simulink model "simulation_with_sensors"  (R2023b)
settings: Solver=VariableStepAuto  StartTime=0.0  StopTime=1000  RelTol=1e-3
values from neighbouring files (symbols this model uses):
  a = R_E+500*1e3    (= 6871000)    [Sensors.m]    (also in sim_with_sensors.m = 6851.22197053; simulation_with_sensors.m = 26584)
  A_313 = ( R_om * R_i * R_OM )'    [simulation_with_sensors.m]
  e = 0    [Sensors.m]    (also in sim_with_sensors.m = 0.00183012221618; simulation_with_sensors.m = 0.00023103)
  H0 = sqrt(g01^2+g11^2+h11^2)*1e-9    [sim_with_sensors.m]    (also in simulation_with_sensors.m)
  I = diag([I1 I2 I3])*1e-9    [sim_with_sensors.m]    (also in simulation_with_sensors.m = diag([100.09 25.1 91.6]))
  i = 1.699980862034725    (= 1.69998086203)    [sim_with_sensors.m]    (also in simulation_with_sensors.m = 0.9601)
  I_inv = inv(I)    [simulation_with_sensors.m]
  incl = deg2rad(11.5)    [sim_with_sensors.m]    (also in simulation_with_sensors.m)
  n = n+1    (= 1)    [Sensors.m]    (also in sim_with_sensors.m = sqrt(mu/a^3); simulation_with_sensors.m = sqrt(astroConstants(13) / a^3))
  omegaE = deg2rad(15)/3600    [sim_with_sensors.m]    (also in simulation_with_sensors.m)
  P = zeros(lenn,lenm)    [Sensors.m]
  s0 = zeros(3,1)    [sim_with_sensors.m]    (also in simulation_with_sensors.m = [0; 0; 0])
  tol = 1e-2    (= 0.01)    [simulation_with_sensors.m]
  w0 = [0.2; 0; 0.2]    [simulation_with_sensors.m]
undefined symbols (not defined in the file or in its folder): A, c1, magnitude, N, n_sun, onesM, onesV, r_Fskew, rho_d, rho_s
libraries: matrix_library x11, dspmathops x10, simulink x3
(part 1 of 2)
settings Model: Creator=danie  LastModifiedBy=danie

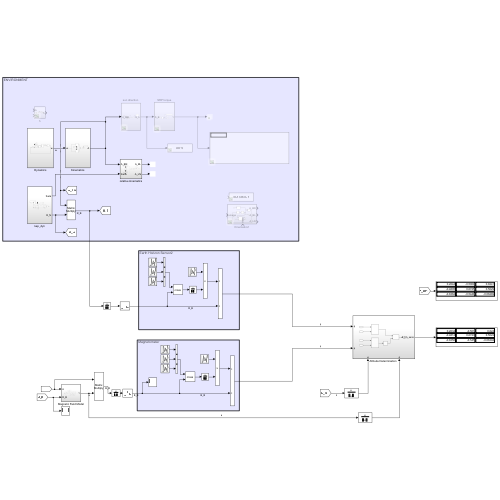
[thumbnail: Simulink's stored preview of the top-level diagram]
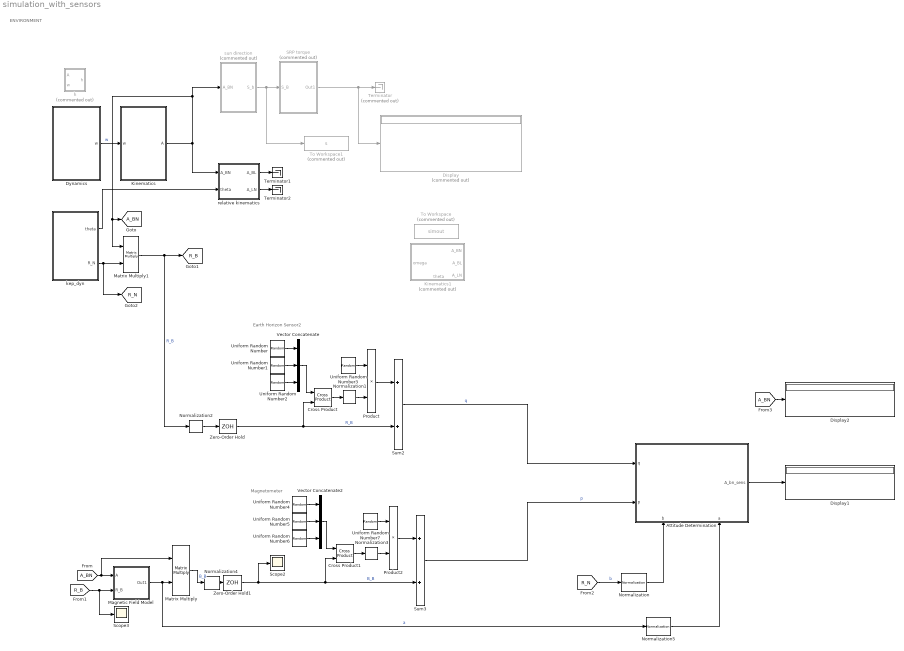
== system simulation_with_sensors ==
  note: ENVIRONMENT
  note: Earth Horizon Sensor2
  note: Magnetometer
  "Attitude Determination  " : Subsystem
      settings: PortSchema="{\"entries\":[{\"content\":{\"sides\":[{\"content\":{\"connectorIds\":[\"In1\",\"In2\"]},\"type\":\"ConnectorPlacement.EquallySpacedRectSide\",\"uuid\":\"730966cf-d0d7-44a0-92f0-b5324480e7cc\"},{\"content\":{\"connectorIds\":[\"Out1\"],\"side\":\"RIGHT\"},\"type\":\"ConnectorPlacement.EquallySpacedRectSide\",\"uuid\":\"c83e6b57-46fe-4a45-9824-d3495e15bf6a\"},{\"content\":{\"side\":\"TOP\"},\"type\":\"ConnectorPlacement.EquallySpacedRectSide\",\"uuid\":\"4938c298-c2b3-45b7-bcb0-70b8132dabc6\"},{\"content\":{\"connectorIds\":[\"In3\",\"In4\"],\"side\":\"BOTTOM\"},\"type\":\"ConnectorPlacement.EquallySpacedRectSide\",\"uuid\":\"6d6a244e-80db-423b-a0a5-9a5face48fcb\"}]},\"type\":\"ConnectorPlacement.EquallySpacedConnector\",\"uuid\":\"7eb6767d-3ff0-4577-86c9-ebc5e763f220\"}],\"packageUris\":[\"http://schema.mathworks.com/mf0/Connector/R2020b\"],\"version\":\"1.0\"}"
  Cross Product : matrix_library/Cross Product
  Cross Product1 : matrix_library/Cross Product
  Display : Display  Commented=on
  Display1 : Display
  Display2 : Display
  Dynamics : Subsystem
  Kinematics : Subsystem
  Kinematics1 : Subsystem  Commented=on
      settings: PortSchema="{\"entries\":[{\"content\":{\"sides\":[{\"content\":{\"connectorIds\":[\"In1\"]},\"type\":\"ConnectorPlacement.EquallySpacedRectSide\",\"uuid\":\"c78567b3-0f16-47a3-80bd-0d4e0067a31f\"},{\"content\":{\"connectorIds\":[\"Out1\",\"Out2\",\"Out3\"],\"side\":\"RIGHT\"},\"type\":\"ConnectorPlacement.EquallySpacedRectSide\",\"uuid\":\"73465dec-5215-44e7-a1cc-75f9f3cf9a64\"},{\"content\":{\"side\":\"TOP\"},\"type\":\"ConnectorPlacement.EquallySpacedRectSide\",\"uuid\":\"3a97d62b-3b72-49ee-88a3-b4c3b7bde741\"},{\"content\":{\"connectorIds\":[\"In2\"],\"side\":\"BOTTOM\"},\"type\":\"ConnectorPlacement.EquallySpacedRectSide\",\"uuid\":\"877f870a-38cc-42df-9514-c8e95f578485\"}]},\"type\":\"ConnectorPlacement.EquallySpacedConnector\",\"uuid\":\"7c502635-8079-4510-841d-e1e17271f078\"}],\"packageUris\":[\"http://schema.mathworks.com/mf0/Connector/R2020b\"],\"version\":\"1.0\"}"
  Magnetic Field Model : Subsystem
  Matrix Multiply : Product  Multiplication=Matrix(*)
  Matrix Multiply1 : Product  Multiplication=Matrix(*)
  Normalization{,1..5} (6 alike) : dspmathops/Normalization  NormType=2-norm  Bias=1e-10  NormOver=Each column  Dimension=1  roundingMode=Floor  overflowMode=off  accumDataTypeStr=Inherit: Same as product output  accumLastDataTypeStr=Inherit: Same as product output  outputDataTypeStr=Inherit: Same as product output  outputMin=[]  outputMax=[]  outputLastDataTypeStr=Inherit: Same as product output
  Product : Product
  Product2 : Product
  SRP torque : Subsystem  Commented=on
  Scope2 : Scope
  Scope3 : Scope
  Sum2 : Sum
  Sum3 : Sum
  Terminator : Terminator  Commented=on
  Terminator1 : Terminator
  Terminator2 : Terminator
  To Workspace : ToWorkspace  Commented=on  VariableName=simout  SaveFormat=Timeseries  SampleTime=-1
  To Workspace1 : ToWorkspace  Commented=on  VariableName=s  SaveFormat=Timeseries  SampleTime=-1
  Uniform Random Number{,1..2,4..6} (6 alike) : UniformRandomNumber
  Uniform Random Number3 : UniformRandomNumber  Minimum=0  Maximum=tan(deg2rad(0.1))
  Uniform Random Number7 : UniformRandomNumber  Minimum=0  Maximum=tan(deg2rad(0.5))
  Vector Concatenate : Concatenate  NumInputs=3
  Vector Concatenate2 : Concatenate  NumInputs=3
  Zero-Order Hold : ZeroOrderHold  SampleTime=1/30
  Zero-Order Hold1 : ZeroOrderHold  SampleTime=1/30
  h : Subsystem  Commented=on
  kep_dyn : Subsystem
  relative kinematics : Subsystem
  "sun direction " : Subsystem  Commented=on
  tag scope: A_BN=global, R_B=global, R_N=global
  wires:
  kep_dyn/2(R_N) -> [R_N], Matrix Multiply1/2
  SRP torque/1(Out1) -> Display/1, Terminator/1
  Dynamics/1(w) -> Kinematics/1(w)  "w"
  "sun direction "/1(S_b) -> SRP torque/1(S_B), To Workspace1/1
  Kinematics/1(A) -> [A_BN], Matrix Multiply1/1, "sun direction "/1(A_BN), relative kinematics/1(A_BN)
  kep_dyn/1(theta) -> relative kinematics/2(theta)
  Sum2/1 -> "Attitude Determination  "/1(q)  "q"
  Normalization1/1 -> Product/2
  Magnetic Field Model/1(Out1) -> Normalization5/1, Matrix Multiply/2  "a"
  Uniform Random Number3/1 -> Product/1
  Uniform Random Number7/1 -> Product2/1
  Uniform Random Number1/1 -> Vector Concatenate/2
  Uniform Random Number5/1 -> Vector Concatenate2/2
  Uniform Random Number4/1 -> Vector Concatenate2/1
  Product/1 -> Sum2/1
  Product2/1 -> Sum3/1
  Zero-Order Hold1/1 -> Cross Product1/2, Sum3/2, Scope2/1  "B_B"
  Vector Concatenate2/1 -> Cross Product1/1
  Normalization3/1 -> Product2/2
  Sum3/1 -> "Attitude Determination  "/2(p)  "p"
  Cross Product1/1 -> Normalization3/1
  Normalization2/1 -> Zero-Order Hold/1
  Zero-Order Hold/1 -> Cross Product/2, Sum2/2  "R_B"
  Uniform Random Number/1 -> Vector Concatenate/1
  Vector Concatenate/1 -> Cross Product/1
  Uniform Random Number2/1 -> Vector Concatenate/3
  Uniform Random Number6/1 -> Vector Concatenate2/3
  Cross Product/1 -> Normalization1/1
  Matrix Multiply1/1 -> [R_B], Normalization2/1  "R_B"
  [A_BN] -> Matrix Multiply/1, Magnetic Field Model/1(A)
  [R_B] -> Scope3/1, Magnetic Field Model/2(R_B)
  relative kinematics/1(A_BL) -> Terminator1/1
  relative kinematics/2(A_LN) -> Terminator2/1
  Normalization4/1 -> Zero-Order Hold1/1
  Matrix Multiply/1 -> Normalization4/1  "B_B"
  [R_N] -> Normalization/1  "b"
  "Attitude Determination  "/1(A_bn_sens) -> Display1/1
  [A_BN] -> Display2/1
  Normalization/1 -> "Attitude Determination  "/3(b)
  Normalization5/1 -> "Attitude Determination  "/4(a)

== system simulation_with_sensors/Attitude Determination   ==
  q : Inport
  p : Inport  Port=2
  b : Inport  Port=3
  a : Inport  Port=4
  Matrix Multiply : Product  Multiplication=Matrix(*)
  S : Subsystem
  Transpose : Math  Operator=transpose
  V : Subsystem
  A_bn_sens : Outport
  wires:
  q/1 -> S/1(q)
  p/1 -> S/2(p)
  a/1 -> V/2(a)
  b/1 -> V/1(b)
  V/1(V) -> Transpose/1
  S/1(S) -> Matrix Multiply/1
  Transpose/1 -> Matrix Multiply/2
  Matrix Multiply/1 -> A_bn_sens/1

== system simulation_with_sensors/Dynamics ==
  Constant : Constant  Value=I
  Constant1 : Constant  Value=-I_inv
  Cross Product : matrix_library/Cross Product
  Integrator : Integrator  InitialCondition=w0
  Product : Product  Multiplication=Matrix(*)
  Product1 : Product  Multiplication=Matrix(*)
  To Workspace : ToWorkspace  VariableName=w  SaveFormat=Timeseries  SampleTime=-1
  w : Outport
  wires:
  Cross Product/1 -> Product1/2
  Constant/1 -> Product/1
  Integrator/1 -> Product/2, w/1, To Workspace/1, Cross Product/1  "w"
  Constant1/1 -> Product1/1
  Product/1 -> Cross Product/2
  Product1/1 -> Integrator/1  "wdot"

== system simulation_with_sensors/Kinematics ==
  w : Inport
  Kinematics 312 : Subsystem
  Kinematics 313 : Subsystem
  Merge : Merge
  NOT : Logic  Operator=NOT  IconShape=distinctive  AllPortsSameDT=off  OutDataTypeStr=boolean
  System switcher : Subsystem
  To Workspace : ToWorkspace  VariableName=A  SaveFormat=Timeseries  SampleTime=-1
  A : Outport
  wires:
  NOT/1 -> Kinematics 313/Enable
  w/1 -> Kinematics 312/1(w), Kinematics 313/1(w)
  System switcher/1(flag) -> Kinematics 312/Enable, NOT/1
  Kinematics 313/1(A) -> Merge/2
  Merge/1 -> A/1, To Workspace/1  "A"
  Kinematics 312/1(A) -> Merge/1

== system simulation_with_sensors/Kinematics1 ==
  omega : Inport
  theta : Inport  Port=2
  Integrator : Integrator  InitialCondition=eye(3)
  Matrix Multiply : Product  Multiplication=Matrix(*)
  om^ : Subsystem
  orthonormalization1 : Subsystem
  relative kinematics : Subsystem
  A_BN : Outport
  A_BL : Outport  Port=2
  A_LN : Outport  Port=3
  wires:
  Integrator/1 -> orthonormalization1/1(A0)
  omega/1 -> om^/1(omega)
  om^/1(" om ^") -> Matrix Multiply/1
  Matrix Multiply/1 -> Integrator/1
  orthonormalization1/1(A) -> relative kinematics/1(A_BN), A_BN/1, Matrix Multiply/2
  relative kinematics/1(A_BL) -> A_BL/1
  theta/1 -> relative kinematics/2(theta)
  relative kinematics/2(A_LN) -> A_LN/1

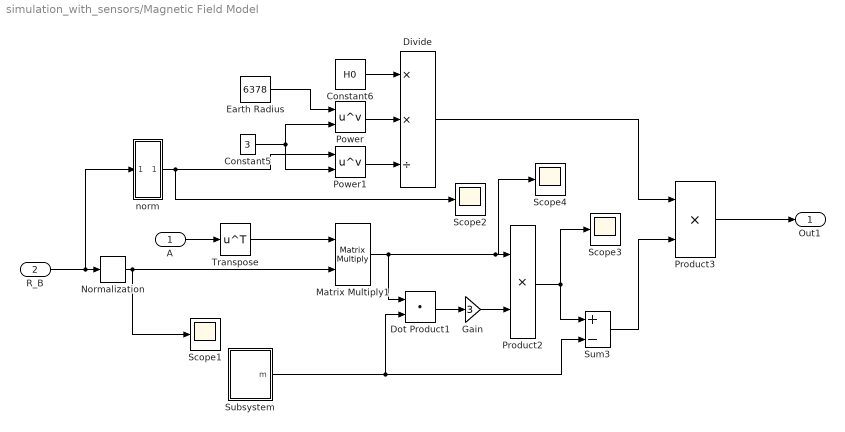
== system simulation_with_sensors/Magnetic Field Model ==
  A : Inport
  R_B : Inport  Port=2
  Constant5 : Constant  Value=3
  Constant6 : Constant  Value=H0
  Divide : Product  Inputs=**/
  Dot Product1 : DotProduct  OutDataTypeStr=Inherit: Inherit via internal rule
  Earth Radius : Constant  Value=6378
  Gain : Gain  Gain=3
  Matrix Multiply1 : Product  Multiplication=Matrix(*)
  Normalization : dspmathops/Normalization  NormType=2-norm  Bias=1e-10  NormOver=Each column  Dimension=1  roundingMode=Floor  overflowMode=off  accumDataTypeStr=Inherit: Same as product output  accumLastDataTypeStr=Inherit: Same as product output  outputDataTypeStr=Inherit: Same as product output  outputMin=[]  outputMax=[]  outputLastDataTypeStr=Inherit: Same as product output
  Power : Math  Operator=pow
  Power1 : Math  Operator=pow
  Product2 : Product
  Product3 : Product
  Scope{1..4} (4 alike) : Scope
  Subsystem : Subsystem
  Sum3 : Sum  Inputs=+-
  Transpose : Math  Operator=transpose
  norm : Subsystem
  Out1 : Outport
  wires:
  Matrix Multiply1/1 -> Scope4/1, Product2/1, Dot Product1/1
  Subsystem/1(m) -> Sum3/2, Dot Product1/2
  R_B/1 -> norm/1(In1), Normalization/1
  Divide/1 -> Product3/1
  Constant5/1 -> Power/2, Power1/2
  Sum3/1 -> Product3/2
  norm/1(Out1) -> Scope2/1, Power1/1
  Dot Product1/1 -> Gain/1
  Gain/1 -> Product2/2
  Product2/1 -> Sum3/1, Scope3/1
  Earth Radius/1 -> Power/1
  Constant6/1 -> Divide/1
  Transpose/1 -> Matrix Multiply1/1
  Power/1 -> Divide/2
  A/1 -> Transpose/1
  Product3/1 -> Out1/1
  Power1/1 -> Divide/3
  Normalization/1 -> Scope1/1, Matrix Multiply1/2

== system simulation_with_sensors/SRP torque ==
  S_B : Inport
  Display : Display
  SRP forces calc : Subsystem
  To Workspace : ToWorkspace  VariableName=SRP_F  SaveFormat=Timeseries  SampleTime=-1
  To Workspace1 : ToWorkspace  VariableName=SRP_T  SaveFormat=Timeseries  SampleTime=-1
  equivalent force system : Subsystem
  Out1 : Outport
  wires:
  equivalent force system/1(Torque) -> Display/1, To Workspace1/1, Out1/1
  equivalent force system/2(Resultant) -> To Workspace/1
  S_B/1 -> SRP forces calc/1(In1)  "SUN DIR."
  SRP forces calc/1(forces) -> equivalent force system/1(Forces)

== system simulation_with_sensors/h ==
  A : Inport
  w : Inport  Port=2
  Constant : Constant  Value=I
  Product1 : Product  Multiplication=Matrix(*)
  Product2 : Product  Multiplication=Matrix(*)
  Transpose : Math  Operator=transpose
  h : Outport
  wires:
  Constant/1 -> Product1/1
  Product2/1 -> h/1  "h"
  Product1/1 -> Product2/2  "h_body"
  A/1 -> Transpose/1
  w/1 -> Product1/2
  Transpose/1 -> Product2/1

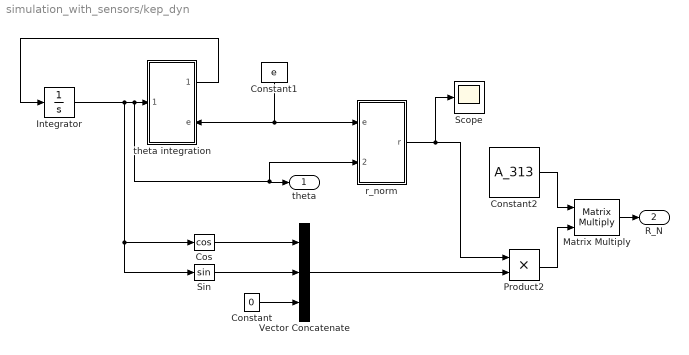
== system simulation_with_sensors/kep_dyn ==
  Constant : Constant  Value=0
  Constant1 : Constant  Value=e
  Constant2 : Constant  Value=A_313
  Cos : Trigonometry  Operator=cos
  Integrator : Integrator
  Matrix Multiply : Product  Multiplication=Matrix(*)
  Product2 : Product
  Scope : Scope
  Sin : Trigonometry
  Vector Concatenate : Concatenate  NumInputs=3
  r_norm : Subsystem
  theta integration : Subsystem
      settings: PortSchema="{\"entries\":[{\"content\":{\"sides\":[{\"content\":{\"connectorIds\":[\"In1\"]},\"type\":\"ConnectorPlacement.EquallySpacedRectSide\",\"uuid\":\"3f1b1ec9-07ed-4eb1-9e41-630dc5613e97\"},{\"content\":{\"connectorIds\":[\"Out1\",\"In2\"],\"side\":\"RIGHT\"},\"type\":\"ConnectorPlacement.EquallySpacedRectSide\",\"uuid\":\"22d0f7bc-714c-4365-a26c-07047ff4be14\"},{\"content\":{\"side\":\"TOP\"},\"type\":\"ConnectorPlacement.EquallySpacedRectSide\",\"uuid\":\"875f7006-d698-4730-93ae-1a7d05f24054\"}]},\"type\":\"ConnectorPlacement.EquallySpacedConnector\",\"uuid\":\"799b65b1-faea-432b-9f3f-2d21984184cd\"}],\"packageUris\":[\"http://schema.mathworks.com/mf0/Connector/R2020b\"],\"version\":\"1.0\"}"
  theta : Outport
  R_N : Outport  Port=2
  wires:
  Integrator/1 -> Sin/1, Cos/1, r_norm/2(theta), theta/1, theta integration/1(theta)
  theta integration/1(theta_dot) -> Integrator/1
  Constant/1 -> Vector Concatenate/3
  Cos/1 -> Vector Concatenate/1
  Constant1/1 -> theta integration/2(e), r_norm/1(e)
  r_norm/1(r) -> Scope/1, Product2/1
  Vector Concatenate/1 -> Product2/2
  Sin/1 -> Vector Concatenate/2
  Constant2/1 -> Matrix Multiply/1
  Product2/1 -> Matrix Multiply/2
  Matrix Multiply/1 -> R_N/1

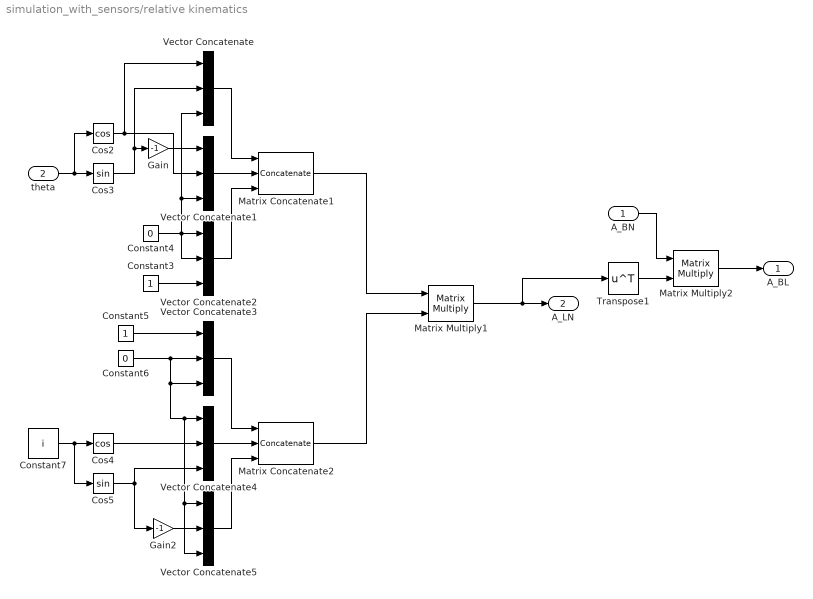
== system simulation_with_sensors/relative kinematics ==
  A_BN : Inport
  theta : Inport  Port=2
  Constant3 : Constant
  Constant4 : Constant  Value=0
  Constant5 : Constant
  Constant6 : Constant  Value=0
  Constant7 : Constant  Value=i
  Cos2 : Trigonometry  Operator=cos
  Cos3 : Trigonometry
  Cos4 : Trigonometry  Operator=cos
  Cos5 : Trigonometry
  Gain : Gain  Gain=-1
  Gain2 : Gain  Gain=-1
  Matrix Concatenate1 : Concatenate  NumInputs=3  Mode=Multidimensional array  ConcatenateDimension=2
  Matrix Concatenate2 : Concatenate  NumInputs=3  Mode=Multidimensional array  ConcatenateDimension=2
  Matrix Multiply1 : Product  Multiplication=Matrix(*)
  Matrix Multiply2 : Product  Multiplication=Matrix(*)
  Transpose1 : Math  Operator=transpose
  Vector Concatenate{,1..5} (6 alike) : Concatenate  NumInputs=3
  A_BL : Outport
  A_LN : Outport  Port=2
  wires:
  Cos2/1 -> Vector Concatenate1/2, Vector Concatenate/1
  Cos3/1 -> Gain/1, Vector Concatenate/2
  Constant4/1 -> Vector Concatenate2/2, Vector Concatenate/3, Vector Concatenate1/3, Vector Concatenate2/1
  Constant3/1 -> Vector Concatenate2/3
  Gain/1 -> Vector Concatenate1/1
  theta/1 -> Cos2/1, Cos3/1
  Vector Concatenate/1 -> Matrix Concatenate1/1
  Vector Concatenate1/1 -> Matrix Concatenate1/2
  Vector Concatenate2/1 -> Matrix Concatenate1/3
  Vector Concatenate5/1 -> Matrix Concatenate2/3
  Constant7/1 -> Cos4/1, Cos5/1
  Vector Concatenate3/1 -> Matrix Concatenate2/1
  Cos5/1 -> Vector Concatenate4/3, Gain2/1
  Vector Concatenate4/1 -> Matrix Concatenate2/2
  Constant5/1 -> Vector Concatenate3/1
  Constant6/1 -> Vector Concatenate5/3, Vector Concatenate5/1, Vector Concatenate4/1, Vector Concatenate3/3, Vector Concatenate3/2
  Cos4/1 -> Vector Concatenate4/2
  Gain2/1 -> Vector Concatenate5/2
  Matrix Concatenate1/1 -> Matrix Multiply1/1
  Matrix Concatenate2/1 -> Matrix Multiply1/2
  Matrix Multiply1/1 -> Transpose1/1, A_LN/1
  A_BN/1 -> Matrix Multiply2/1
  Transpose1/1 -> Matrix Multiply2/2
  Matrix Multiply2/1 -> A_BL/1

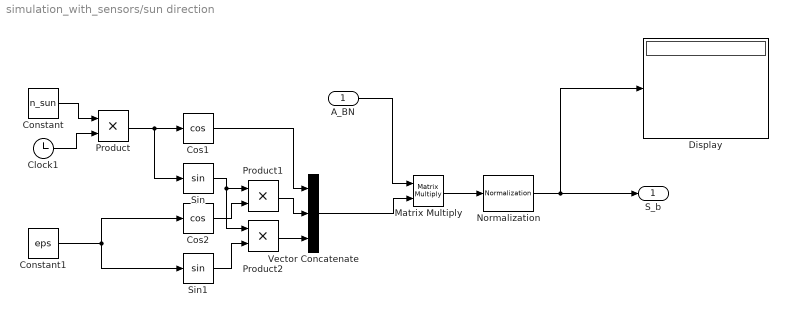
== system simulation_with_sensors/sun direction  ==
  A_BN : Inport
  Clock1 : Clock
  Constant : Constant  Value=n_sun
  Constant1 : Constant  Value=eps
  Cos1 : Trigonometry  Operator=cos
  Cos2 : Trigonometry  Operator=cos
  Display : Display
  Matrix Multiply : Product  Multiplication=Matrix(*)
  Normalization : dspmathops/Normalization  NormType=Squared 2-norm  Bias=1e-10  NormOver=Each column  Dimension=1  roundingMode=Floor  overflowMode=off  accumDataTypeStr=Inherit: Same as product output  accumLastDataTypeStr=Inherit: Same as product output  outputDataTypeStr=Inherit: Same as product output  outputMin=[]  outputMax=[]  outputLastDataTypeStr=Inherit: Same as product output
  Product : Product
  Product1 : Product
  Product2 : Product
  Sin : Trigonometry
  Sin1 : Trigonometry
  Vector Concatenate : Concatenate  NumInputs=3
  S_b : Outport
  wires:
  Constant/1 -> Product/1
  Clock1/1 -> Product/2
  Product/1 -> Sin/1, Cos1/1
  Constant1/1 -> Sin1/1, Cos2/1
  Sin/1 -> Product2/1, Product1/1
  Cos2/1 -> Product1/2
  Sin1/1 -> Product2/2
  Cos1/1 -> Vector Concatenate/1
  Product1/1 -> Vector Concatenate/2
  Product2/1 -> Vector Concatenate/3
  Matrix Multiply/1 -> Normalization/1
  A_BN/1 -> Matrix Multiply/1
  Normalization/1 -> Display/1, S_b/1
  Vector Concatenate/1 -> Matrix Multiply/2

== system simulation_with_sensors/Attitude Determination  /S ==
  q : Inport
  p : Inport  Port=2
  Cross Product : matrix_library/Cross Product
  Cross Product1 : matrix_library/Cross Product
  Matrix Concatenate : Concatenate  NumInputs=3  Mode=Multidimensional array  ConcatenateDimension=2
  Normalization : dspmathops/Normalization  NormType=2-norm  Bias=1e-10  NormOver=Each column  Dimension=1  roundingMode=Floor  overflowMode=off  accumDataTypeStr=Inherit: Same as product output  accumLastDataTypeStr=Inherit: Same as product output  outputDataTypeStr=Inherit: Same as product output  outputMin=[]  outputMax=[]  outputLastDataTypeStr=Inherit: Same as product output
  S : Outport
  wires:
  p/1 -> Matrix Concatenate/1, Cross Product/1, Cross Product1/1
  q/1 -> Cross Product/2
  Cross Product/1 -> Normalization/1
  Normalization/1 -> Matrix Concatenate/2, Cross Product1/2
  Matrix Concatenate/1 -> S/1
  Cross Product1/1 -> Matrix Concatenate/3

== system simulation_with_sensors/Attitude Determination  /V ==
  b : Inport
  a : Inport  Port=2
  Cross Product : matrix_library/Cross Product
  Cross Product1 : matrix_library/Cross Product
  Matrix Concatenate : Concatenate  NumInputs=3  Mode=Multidimensional array  ConcatenateDimension=2
  Normalization : dspmathops/Normalization  NormType=2-norm  Bias=1e-10  NormOver=Each column  Dimension=1  roundingMode=Floor  overflowMode=off  accumDataTypeStr=Inherit: Same as product output  accumLastDataTypeStr=Inherit: Same as product output  outputDataTypeStr=Inherit: Same as product output  outputMin=[]  outputMax=[]  outputLastDataTypeStr=Inherit: Same as product output
  V : Outport
  wires:
  Cross Product1/1 -> Matrix Concatenate/3
  Matrix Concatenate/1 -> V/1
  Normalization/1 -> Cross Product1/2, Matrix Concatenate/2
  Cross Product/1 -> Normalization/1
  b/1 -> Cross Product/2
  a/1 -> Cross Product1/1, Cross Product/1, Matrix Concatenate/1

== system simulation_with_sensors/Kinematics/Kinematics 312 ==
  w : Inport
  Enable : EnablePort  StatesWhenEnabling=reset
  A - s_312 : Subsystem
  Euler angles : Subsystem
  IC : InitialCondition  Value=s0
  s_312 - A : Subsystem
  s_313 - A : Subsystem
  A : Outport
  wires:
  s_312 - A/1(A) -> A/1  "A"
  Euler angles/1(s) -> s_312 - A/1(s)  "s"
  w/1 -> Euler angles/1(w)
  IC/1 -> Euler angles/2(s0)
  A - s_312/1(s) -> IC/1
  s_313 - A/1(A) -> A - s_312/1(A)
  [s_313] -> s_313 - A/1(s)

== system simulation_with_sensors/Kinematics/Kinematics 313 ==
  w : Inport
  Enable : EnablePort  StatesWhenEnabling=reset
  A - s_313 : Subsystem
  Euler angles : Subsystem
  s_312 - A : Subsystem
  s_313 - A : Subsystem
  A : Outport
  wires:
  w/1 -> Euler angles/1(w)
  Euler angles/1(s) -> s_313 - A/1(s)
  s_313 - A/1(A) -> A/1
  A - s_313/1(s) -> Euler angles/2(s0)
  s_312 - A/1(A) -> A - s_313/1(A)
  [s_312] -> s_312 - A/1(s)

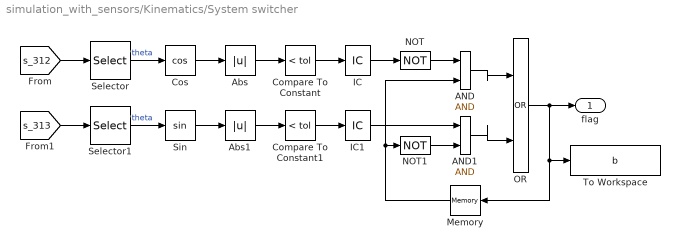
== system simulation_with_sensors/Kinematics/System switcher ==
  AND : Logic  IconShape=distinctive  AllPortsSameDT=off  OutDataTypeStr=boolean
  AND1 : Logic  IconShape=distinctive  AllPortsSameDT=off  OutDataTypeStr=boolean
  Abs : Abs  SaturateOnIntegerOverflow=off
  Abs1 : Abs  SaturateOnIntegerOverflow=off
  Compare To Constant : simulink/Logic and Bit Operations/Compare To Constant  relop=<  const=tol  OutDataTypeStr=boolean
  Compare To Constant1 : simulink/Logic and Bit Operations/Compare To Constant  relop=<  const=tol  OutDataTypeStr=boolean
  Cos : Trigonometry  Operator=cos
  IC : InitialCondition  Value=0
  IC1 : InitialCondition  Value=0
  Memory : Memory  InitialCondition=1
  NOT : Logic  Operator=NOT  IconShape=distinctive  AllPortsSameDT=off  OutDataTypeStr=boolean
  NOT1 : Logic  Operator=NOT  IconShape=distinctive  AllPortsSameDT=off  OutDataTypeStr=boolean
  OR : Logic  Operator=OR  IconShape=distinctive  AllPortsSameDT=off  OutDataTypeStr=boolean
  Selector : Selector  InputPortWidth=3  IndexOptions=Index vector (dialog)  Indices=2  OutputSizes=1
  Selector1 : Selector  InputPortWidth=3  IndexOptions=Index vector (dialog)  Indices=2  OutputSizes=1
  Sin : Trigonometry
  To Workspace : ToWorkspace  VariableName=b  SaveFormat=Timeseries  SampleTime=-1
  flag : Outport
  wires:
  Cos/1 -> Abs/1
  [s_312] -> Selector/1
  Compare To Constant/1 -> IC/1
  Selector1/1 -> Sin/1  "theta"
  Abs/1 -> Compare To Constant/1
  Compare To Constant1/1 -> IC1/1
  Selector/1 -> Cos/1  "theta"
  Abs1/1 -> Compare To Constant1/1
  Sin/1 -> Abs1/1
  [s_313] -> Selector1/1
  IC/1 -> NOT/1
  NOT/1 -> AND/1
  AND/1 -> OR/1
  NOT1/1 -> AND1/2
  IC1/1 -> AND1/1
  AND1/1 -> OR/2
  OR/1 -> To Workspace/1, Memory/1, flag/1
  Memory/1 -> AND/2, NOT1/1

== system simulation_with_sensors/Kinematics1/om^ ==
  omega : Inport
  Constant : Constant  Value=[1; 0; 0]
  Constant1 : Constant  Value=[0; 1; 0]
  Constant2 : Constant  Value=[0; 0; 1]
  Cross Product : matrix_library/Cross Product
  Cross Product1 : matrix_library/Cross Product
  Cross Product2 : matrix_library/Cross Product
  Matrix Concatenate : Concatenate  NumInputs=3  Mode=Multidimensional array  ConcatenateDimension=2
  " om ^" : Outport
  wires:
  Matrix Concatenate/1 -> " om ^"/1
  Cross Product2/1 -> Matrix Concatenate/3
  Cross Product1/1 -> Matrix Concatenate/2
  Cross Product/1 -> Matrix Concatenate/1
  Constant/1 -> Cross Product/1
  Constant1/1 -> Cross Product1/1
  Constant2/1 -> Cross Product2/1
  omega/1 -> Cross Product/2, Cross Product1/2, Cross Product2/2

== system simulation_with_sensors/Kinematics1/orthonormalization1 ==
  A0 : Inport
  Gain : Gain  Gain=3/2
  Gain1 : Gain  Gain=1/2
  Matrix Multiply : Product  Inputs=3  Multiplication=Matrix(*)
  Sum : Sum  Inputs=-|+
  Transpose : matrix_library/Transpose
  A : Outport
  wires:
  Sum/1 -> A/1
  Gain1/1 -> Sum/1
  Matrix Multiply/1 -> Gain1/1
  Transpose/1 -> Matrix Multiply/2
  Gain/1 -> Sum/2
  A0/1 -> Gain/1, Matrix Multiply/3, Transpose/1, Matrix Multiply/1

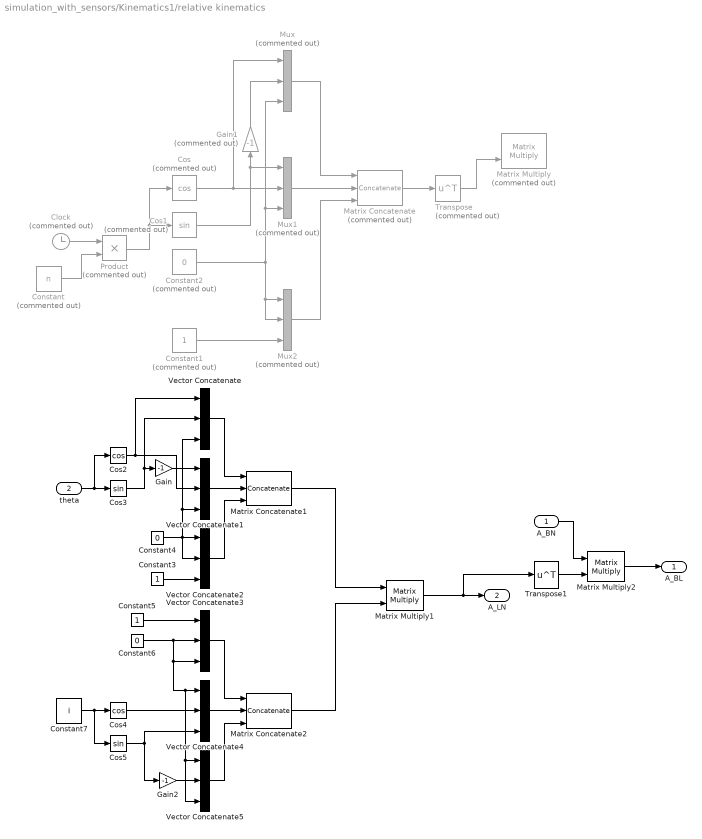
== system simulation_with_sensors/Kinematics1/relative kinematics ==
  A_BN : Inport
  theta : Inport  Port=2
  Clock : Clock  Commented=on
  Constant : Constant  Commented=on  Value=n
  Constant1 : Constant  Commented=on
  Constant2 : Constant  Commented=on  Value=0
  Constant3 : Constant
  Constant4 : Constant  Value=0
  Constant5 : Constant
  Constant6 : Constant  Value=0
  Constant7 : Constant  Value=i
  Cos : Trigonometry  Commented=on  Operator=cos
  Cos1 : Trigonometry  Commented=on
  Cos2 : Trigonometry  Operator=cos
  Cos3 : Trigonometry
  Cos4 : Trigonometry  Operator=cos
  Cos5 : Trigonometry
  Gain : Gain  Gain=-1
  Gain1 : Gain  Commented=on  Gain=-1
  Gain2 : Gain  Gain=-1
  Matrix Concatenate : Concatenate  Commented=on  NumInputs=3  Mode=Multidimensional array  ConcatenateDimension=2
  Matrix Concatenate1 : Concatenate  NumInputs=3  Mode=Multidimensional array  ConcatenateDimension=2
  Matrix Concatenate2 : Concatenate  NumInputs=3  Mode=Multidimensional array  ConcatenateDimension=2
  Matrix Multiply : Product  Commented=on  Multiplication=Matrix(*)
  Matrix Multiply1 : Product  Multiplication=Matrix(*)
  Matrix Multiply2 : Product  Multiplication=Matrix(*)
  Mux : Mux  Commented=on  Inputs=3
  Mux1 : Mux  Commented=on  Inputs=3
  Mux2 : Mux  Commented=on  Inputs=3
  Product : Product  Commented=on
  Transpose : Math  Commented=on  Operator=transpose
  Transpose1 : Math  Operator=transpose
  Vector Concatenate{,1..5} (6 alike) : Concatenate  NumInputs=3
  A_BL : Outport
  A_LN : Outport  Port=2
  wires:
  Product/1 -> Cos1/1, Cos/1
  Cos/1 -> Mux1/2, Mux/1
  Cos1/1 -> Gain1/1, Mux1/1
  Constant2/1 -> Mux1/3, Mux/3, Mux2/2, Mux2/1
  Gain1/1 -> Mux/2
  Constant1/1 -> Mux2/3
  Mux/1 -> Matrix Concatenate/1
  Mux1/1 -> Matrix Concatenate/2
  Mux2/1 -> Matrix Concatenate/3
  Matrix Concatenate/1 -> Transpose/1
  Transpose/1 -> Matrix Multiply/2
  Clock/1 -> Product/1
  Constant/1 -> Product/2
  Cos2/1 -> Vector Concatenate1/2, Vector Concatenate/1
  Cos3/1 -> Gain/1, Vector Concatenate/2
  Constant4/1 -> Vector Concatenate2/2, Vector Concatenate/3, Vector Concatenate1/3, Vector Concatenate2/1
  Constant3/1 -> Vector Concatenate2/3
  Gain/1 -> Vector Concatenate1/1
  theta/1 -> Cos2/1, Cos3/1
  Vector Concatenate/1 -> Matrix Concatenate1/1
  Vector Concatenate1/1 -> Matrix Concatenate1/2
  Vector Concatenate2/1 -> Matrix Concatenate1/3
  Vector Concatenate5/1 -> Matrix Concatenate2/3
  Constant7/1 -> Cos4/1, Cos5/1
  Vector Concatenate3/1 -> Matrix Concatenate2/1
  Cos5/1 -> Vector Concatenate4/3, Gain2/1
  Vector Concatenate4/1 -> Matrix Concatenate2/2
  Constant5/1 -> Vector Concatenate3/1
  Constant6/1 -> Vector Concatenate5/3, Vector Concatenate5/1, Vector Concatenate4/1, Vector Concatenate3/3, Vector Concatenate3/2
  Cos4/1 -> Vector Concatenate4/2
  Gain2/1 -> Vector Concatenate5/2
  Matrix Concatenate1/1 -> Matrix Multiply1/1
  Matrix Concatenate2/1 -> Matrix Multiply1/2
  Matrix Multiply1/1 -> Transpose1/1, A_LN/1
  A_BN/1 -> Matrix Multiply2/1
  Transpose1/1 -> Matrix Multiply2/2
  Matrix Multiply2/1 -> A_BL/1

== system simulation_with_sensors/Magnetic Field Model/Subsystem ==
  Clock : Clock
  Constant : Constant  Value=incl
  Constant1 : Constant  Value=omegaE
  Cos : Trigonometry  Operator=cos
  Cos1 : Trigonometry  Operator=cos
  Product : Product
  Product1 : Product
  Product2 : Product
  Sin : Trigonometry
  Sin1 : Trigonometry
  Vector Concatenate : Concatenate  NumInputs=3
  m : Outport
  wires:
  Constant/1 -> Cos/1, Sin/1
  Clock/1 -> Product/1
  Constant1/1 -> Product/2
  Product/1 -> Sin1/1, Cos1/1
  Cos1/1 -> Product1/1
  Sin/1 -> Product2/2, Product1/2
  Sin1/1 -> Product2/1
  Product1/1 -> Vector Concatenate/1
  Product2/1 -> Vector Concatenate/2
  Cos/1 -> Vector Concatenate/3
  Vector Concatenate/1 -> m/1

== system simulation_with_sensors/Magnetic Field Model/norm ==
  In1 : Inport
  Dot Product : DotProduct  OutDataTypeStr=Inherit: Inherit via internal rule
  Sqrt : Sqrt
  Out1 : Outport
  wires:
  In1/1 -> Dot Product/2, Dot Product/1
  Dot Product/1 -> Sqrt/1
  Sqrt/1 -> Out1/1

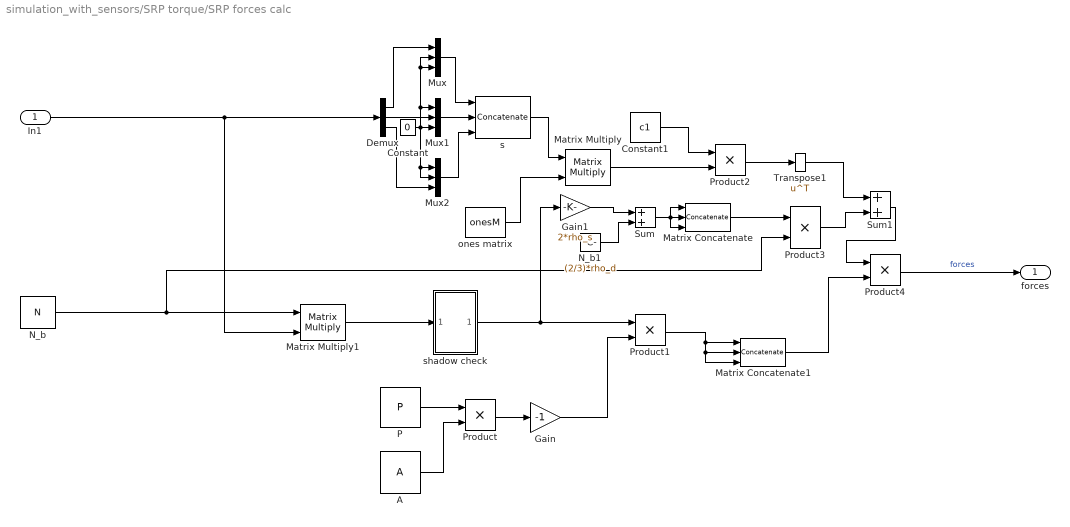
== system simulation_with_sensors/SRP torque/SRP forces calc ==
  In1 : Inport
  A : Constant  Value=A
  Constant : Constant  Value=0
  Constant1 : Constant  Value=c1
  Demux : Demux  Outputs=3
  Gain : Gain  Gain=-1
  Gain1 : Gain  Gain=2*rho_s
  Matrix Concatenate : Concatenate  NumInputs=3  Mode=Multidimensional array  ConcatenateDimension=2
  Matrix Concatenate1 : Concatenate  NumInputs=3  Mode=Multidimensional array  ConcatenateDimension=2
  Matrix Multiply : Product  Multiplication=Matrix(*)
  Matrix Multiply1 : Product  Multiplication=Matrix(*)
  Mux : Mux  Inputs=3
  Mux1 : Mux  Inputs=3
  Mux2 : Mux  Inputs=3
  N_b : Constant  Value=N
  N_b1 : Constant  Value=(2/3)*rho_d
  P : Constant  Value=P
  Product{,1..4} (5 alike) : Product
  Sum : Sum
  Sum1 : Sum
  Transpose1 : Math  Operator=transpose
  ones matrix : Constant  Value=onesM
  "s " : Concatenate  NumInputs=3  Mode=Multidimensional array  ConcatenateDimension=2
  shadow check : Subsystem
  forces : Outport
  wires:
  Product2/1 -> Transpose1/1
  Matrix Multiply/1 -> Product2/2
  N_b/1 -> Product3/2, Matrix Multiply1/1
  P/1 -> Product/1
  ones matrix/1 -> Matrix Multiply/2
  Mux/1 -> "s "/1
  Sum1/1 -> Product4/1
  Mux2/1 -> "s "/3
  Matrix Multiply1/1 -> shadow check/1(In1)
  Gain1/1 -> Sum/1
  Constant/1 -> Mux2/2, Mux2/1, Mux/2, Mux/3, Mux1/1, Mux1/3
  Demux/1 -> Mux/1
  N_b1/1 -> Sum/2
  Product3/1 -> Sum1/2
  Demux/3 -> Mux2/3
  Product1/1 -> Matrix Concatenate1/3, Matrix Concatenate1/2, Matrix Concatenate1/1
  In1/1 -> Demux/1, Matrix Multiply1/2
  Product/1 -> Gain/1
  Matrix Concatenate/1 -> Product3/1
  A/1 -> Product/2
  shadow check/1(Out1) -> Product1/1, Gain1/1
  Demux/2 -> Mux1/2
  Mux1/1 -> "s "/2
  Sum/1 -> Matrix Concatenate/3, Matrix Concatenate/1, Matrix Concatenate/2
  Gain/1 -> Product1/2
  Matrix Concatenate1/1 -> Product4/2
  "s "/1 -> Matrix Multiply/1
  Transpose1/1 -> Sum1/1
  Constant1/1 -> Product2/1
  Product4/1 -> forces/1  "forces"

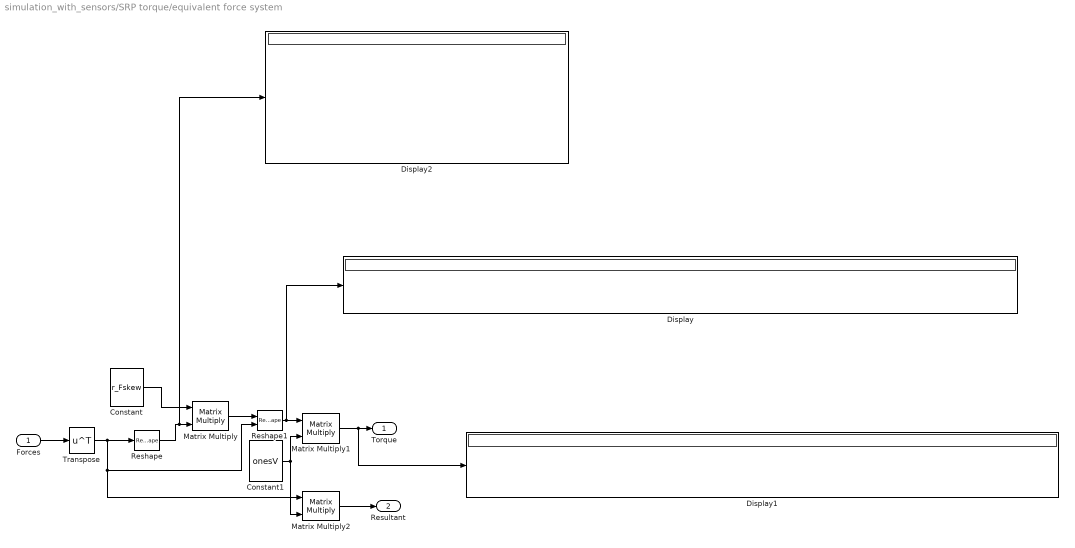
== system simulation_with_sensors/SRP torque/equivalent force system ==
  Forces : Inport
  Constant : Constant  Value=r_Fskew
  Constant1 : Constant  Value=onesV
  Display : Display
  Display1 : Display
  Display2 : Display
  Matrix Multiply : Product  Multiplication=Matrix(*)
  Matrix Multiply1 : Product  Multiplication=Matrix(*)
  Matrix Multiply2 : Product  Multiplication=Matrix(*)
  Reshape : Reshape  OutputDimensionality=Column vector (2-D)
  Reshape1 : Reshape  OutputDimensionality=Derive from reference input port
  Transpose : Math  Operator=transpose
  Torque : Outport
  Resultant : Outport  Port=2
  wires:
  Forces/1 -> Transpose/1
  Reshape/1 -> Display2/1, Matrix Multiply/2
  Constant/1 -> Matrix Multiply/1
  Transpose/1 -> Reshape/1, Matrix Multiply2/1, Reshape1/2
  Matrix Multiply/1 -> Reshape1/1
  Matrix Multiply1/1 -> Display1/1, Torque/1
  Reshape1/1 -> Display/1, Matrix Multiply1/1
  Constant1/1 -> Matrix Multiply1/2, Matrix Multiply2/2
  Matrix Multiply2/1 -> Resultant/1

== system simulation_with_sensors/kep_dyn/r_norm ==
  e : Inport
  theta : Inport  Port=2
  Constant : Constant  Value=a
  Constant1 : Constant
  Cos : Trigonometry  Operator=cos
  Divide : Product  Inputs=*/
  Power : Math  Operator=magnitude^2
  Product : Product
  Product1 : Product
  Sum : Sum  Inputs=+-
  Sum2 : Sum
  r : Outport
  wires:
  e/1 -> Product1/2, Power/1
  Power/1 -> Sum/2
  Constant1/1 -> Sum2/2, Sum/1
  Sum/1 -> Product/2
  Constant/1 -> Product/1
  theta/1 -> Cos/1
  Cos/1 -> Product1/1
  Product1/1 -> Sum2/1
  Divide/1 -> r/1
  Sum2/1 -> Divide/2
  Product/1 -> Divide/1

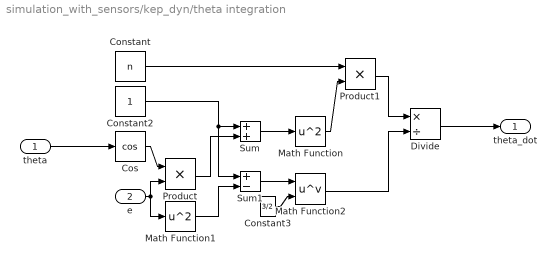
== system simulation_with_sensors/kep_dyn/theta integration ==
  theta : Inport
  e : Inport  Port=2
  Constant : Constant  Value=n
  Constant2 : Constant
  Constant3 : Constant  Value=3/2
  Cos : Trigonometry  Operator=cos
  Divide : Product  Inputs=*/
  Math Function : Math  Operator=square
  Math Function1 : Math  Operator=square
  Math Function2 : Math  Operator=pow
  Product : Product
  Product1 : Product
  Sum : Sum
  Sum1 : Sum  Inputs=+-
  theta_dot : Outport
  wires:
  Product1/1 -> Divide/1
  Product/1 -> Sum/2
  Math Function2/1 -> Divide/2
  Sum1/1 -> Math Function2/1
  Constant2/1 -> Sum1/1, Sum/1
  Math Function1/1 -> Sum1/2
  e/1 -> Product/2, Math Function1/1
  Constant3/1 -> Math Function2/2
  Constant/1 -> Product1/1
  Sum/1 -> Math Function/1
  Math Function/1 -> Product1/2
  Cos/1 -> Product/1
  theta/1 -> Cos/1
  Divide/1 -> theta_dot/1

== system simulation_with_sensors/Kinematics/Kinematics 312/A - s_312 ==
  A : Inport
  Asin : Trigonometry  Operator=asin
  Atan1 : Trigonometry  Operator=atan2
  Atan2 : Trigonometry  Operator=atan2
  Gain : Gain  Gain=-1
  Gain1 : Gain  Gain=-1
  Mux : Mux  Inputs=3
  Selector : Selector  NumberOfDimensions=2  InputPortWidth=3  IndexOptions=Index vector (dialog),Index vector (dialog)  Indices=2,1  OutputSizes=1,1
  Selector1 : Selector  NumberOfDimensions=2  InputPortWidth=3  IndexOptions=Index vector (dialog),Index vector (dialog)  Indices=2,2  OutputSizes=1,1
  Selector2 : Selector  NumberOfDimensions=2  InputPortWidth=3  IndexOptions=Index vector (dialog),Index vector (dialog)  Indices=2,3  OutputSizes=1,1
  Selector3 : Selector  NumberOfDimensions=2  InputPortWidth=3  IndexOptions=Index vector (dialog),Index vector (dialog)  Indices=1,3  OutputSizes=1,1
  Selector4 : Selector  NumberOfDimensions=2  InputPortWidth=3  IndexOptions=Index vector (dialog),Index vector (dialog)  Indices=3,3  OutputSizes=1,1
  s : Outport
  wires:
  Mux/1 -> s/1
  Selector4/1 -> Atan1/2  "a33"
  Atan1/1 -> Mux/3  "psi"
  Atan2/1 -> Mux/1  "phi"
  A/1 -> Selector2/1, Selector1/1, Selector/1, Selector3/1, Selector4/1
  Selector2/1 -> Asin/1  "a23"
  Selector3/1 -> Gain1/1  "a13"
  Selector1/1 -> Atan2/2  "a22"
  Selector/1 -> Gain/1  "a21"
  Asin/1 -> Mux/2  "theta"
  Gain/1 -> Atan2/1
  Gain1/1 -> Atan1/1

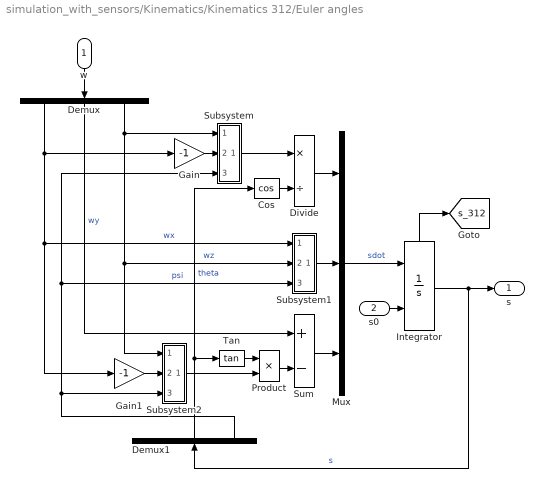
== system simulation_with_sensors/Kinematics/Kinematics 312/Euler angles ==
  w : Inport
  s0 : Inport  Port=2
  Cos : Trigonometry  Operator=cos
  Demux : Demux  Outputs=3
  Demux1 : Demux  Outputs=3
  Divide : Product  Inputs=*/
  Gain : Gain  Gain=-1
  Gain1 : Gain  Gain=-1
  Integrator : Integrator  InitialConditionSource=external  InitialCondition=s0  WrapState=on  WrappedStateUpperValue=2*pi  WrappedStateLowerValue=0  ShowStatePort=on
  Mux : Mux  Inputs=3
  Product : Product
  Subsystem : Subsystem
  Subsystem1 : Subsystem
  Subsystem2 : Subsystem
  Sum : Sum  Inputs=+-
  Tan : Trigonometry  Operator=tan
  s : Outport
  tag scope: s_312=global
  wires:
  w/1 -> Demux/1
  Integrator/1 -> Demux1/1, s/1  "s"
  Demux/3 -> Subsystem2/1(In1), Subsystem1/2(In2), Subsystem/1(In1)  "wz"
  Gain/1 -> Subsystem/2(In2)
  Demux/1 -> Gain1/1, Subsystem1/1(In1), Gain/1  "wx"
  Demux1/3 -> Subsystem2/3(In3), Subsystem1/3(In3), Subsystem/3(In3)  "psi"
  Subsystem/1(Out1) -> Divide/1
  Cos/1 -> Divide/2
  Demux1/2 -> Cos/1, Tan/1  "theta"
  Divide/1 -> Mux/1
  Subsystem1/1(Out1) -> Mux/2
  Gain1/1 -> Subsystem2/2(In2)
  Tan/1 -> Product/1
  Subsystem2/1(Out1) -> Product/2
  Product/1 -> Sum/2
  Demux/2 -> Sum/1  "wy"
  Sum/1 -> Mux/3
  Mux/1 -> Integrator/1  "sdot"
  s0/1 -> Integrator/2
  Integrator/State -> [s_312]

== system simulation_with_sensors/Kinematics/Kinematics 312/s_312 - A ==
  s : Inport
  Demux : Demux  Outputs=3
  Product : Product  Inputs=3  Multiplication=Matrix(*)
  R1 : Subsystem
  R2 : Subsystem
  R3 : Subsystem
  A : Outport
  wires:
  s/1 -> Demux/1  "s"
  R1/1(R1) -> Product/2
  R3/1(R3) -> Product/3
  R2/1(R2) -> Product/1
  Product/1 -> A/1
  Demux/2 -> R1/1(x)  "theta"
  Demux/1 -> R3/1(x)  "phi"
  Demux/3 -> R2/1(x)  "psi"

== system simulation_with_sensors/Kinematics/Kinematics 312/s_313 - A ==
  s : Inport
  Demux : Demux  Outputs=3
  Product : Product  Inputs=3  Multiplication=Matrix(*)
  R1 : Subsystem
  R3_1 : Subsystem
  R3_2 : Subsystem
  A : Outport
  wires:
  Demux/3 -> R3_2/1(x)  "psi"
  Demux/1 -> R3_1/1(x)  "phi"
  Demux/2 -> R1/1(x)  "theta"
  Product/1 -> A/1
  R1/1(R1) -> Product/2
  s/1 -> Demux/1  "s"
  R3_1/1(R3) -> Product/3
  R3_2/1(R3) -> Product/1

== system simulation_with_sensors/Kinematics/Kinematics 313/A - s_313 ==
  A : Inport
  Acos : Trigonometry  Operator=acos
  Atan1 : Trigonometry  Operator=atan2
  Atan2 : Trigonometry  Operator=atan2
  Gain : Gain  Gain=-1
  Mux : Mux  Inputs=3
  Selector : Selector  NumberOfDimensions=2  InputPortWidth=3  IndexOptions=Index vector (dialog),Index vector (dialog)  Indices=3,1  OutputSizes=1,1
  Selector1 : Selector  NumberOfDimensions=2  InputPortWidth=3  IndexOptions=Index vector (dialog),Index vector (dialog)  Indices=3,2  OutputSizes=1,1
  Selector2 : Selector  NumberOfDimensions=2  InputPortWidth=3  IndexOptions=Index vector (dialog),Index vector (dialog)  Indices=3,3  OutputSizes=1,1
  Selector3 : Selector  NumberOfDimensions=2  InputPortWidth=3  IndexOptions=Index vector (dialog),Index vector (dialog)  Indices=1,3  OutputSizes=1,1
  Selector4 : Selector  NumberOfDimensions=2  InputPortWidth=3  IndexOptions=Index vector (dialog),Index vector (dialog)  Indices=2,3  OutputSizes=1,1
  s : Outport
  wires:
  Acos/1 -> Mux/2  "theta"
  Selector/1 -> Atan2/1  "a31"
  Selector1/1 -> Gain/1  "a32"
  Selector3/1 -> Atan1/1  "a13"
  Selector2/1 -> Acos/1  "a33"
  A/1 -> Selector4/1, Selector3/1, Selector/1, Selector1/1, Selector2/1
  Atan2/1 -> Mux/1  "phi"
  Atan1/1 -> Mux/3  "psi"
  Gain/1 -> Atan2/2
  Selector4/1 -> Atan1/2  "a23"
  Mux/1 -> s/1

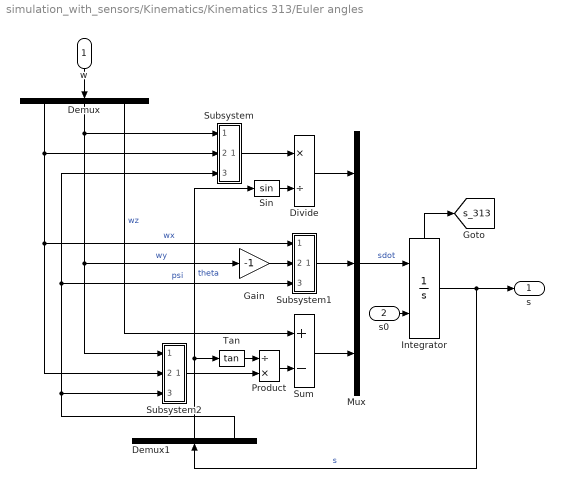
== system simulation_with_sensors/Kinematics/Kinematics 313/Euler angles ==
  w : Inport
  s0 : Inport  Port=2
  Demux : Demux  Outputs=3
  Demux1 : Demux  Outputs=3
  Divide : Product  Inputs=*/
  Gain : Gain  Gain=-1
  Integrator : Integrator  InitialConditionSource=external  InitialCondition=s0  WrapState=on  WrappedStateUpperValue=2*pi  WrappedStateLowerValue=0  ShowStatePort=on
  Mux : Mux  Inputs=3
  Product : Product  Inputs=/*
  Sin : Trigonometry
  Subsystem : Subsystem
  Subsystem1 : Subsystem
  Subsystem2 : Subsystem
  Sum : Sum  Inputs=+-
  Tan : Trigonometry  Operator=tan
  s : Outport
  tag scope: s_313=global
  wires:
  Mux/1 -> Integrator/1  "sdot"
  Sum/1 -> Mux/3
  Demux/2 -> Subsystem/1(In1), Subsystem2/1(In1), Gain/1  "wy"
  Product/1 -> Sum/2
  Subsystem2/1(Out1) -> Product/2
  Tan/1 -> Product/1
  Subsystem1/1(Out1) -> Mux/2
  Divide/1 -> Mux/1
  Demux1/2 -> Sin/1, Tan/1  "theta"
  Subsystem/1(Out1) -> Divide/1
  Demux1/3 -> Subsystem/3(In3), Subsystem1/3(In3), Subsystem2/3(In3)  "psi"
  Demux/1 -> Subsystem2/2(In2), Subsystem1/1(In1), Subsystem/2(In2)  "wx"
  Demux/3 -> Sum/1  "wz"
  Integrator/1 -> Demux1/1, s/1  "s"
  w/1 -> Demux/1
  Sin/1 -> Divide/2
  Gain/1 -> Subsystem1/2(In2)
  s0/1 -> Integrator/2
  Integrator/State -> [s_313]

== system simulation_with_sensors/Kinematics/Kinematics 313/s_312 - A ==
  s : Inport
  Demux : Demux  Outputs=3
  Product : Product  Inputs=3  Multiplication=Matrix(*)
  R1 : Subsystem
  R2 : Subsystem
  R3 : Subsystem
  A : Outport
  wires:
  s/1 -> Demux/1  "s"
  R1/1(R1) -> Product/2
  R3/1(R3) -> Product/3
  R2/1(R2) -> Product/1
  Product/1 -> A/1
  Demux/2 -> R1/1(x)  "theta"
  Demux/1 -> R3/1(x)  "phi"
  Demux/3 -> R2/1(x)  "psi"

== system simulation_with_sensors/Kinematics/Kinematics 313/s_313 - A ==
  s : Inport
  Demux : Demux  Outputs=3
  Product : Product  Inputs=3  Multiplication=Matrix(*)
  R1 : Subsystem
  R3_1 : Subsystem
  R3_2 : Subsystem
  A : Outport
  wires:
  Demux/3 -> R3_2/1(x)  "psi"
  Demux/1 -> R3_1/1(x)  "phi"
  Demux/2 -> R1/1(x)  "theta"
  Product/1 -> A/1
  R1/1(R1) -> Product/2
  s/1 -> Demux/1  "s"
  R3_1/1(R3) -> Product/3
  R3_2/1(R3) -> Product/1

== system simulation_with_sensors/SRP torque/SRP forces calc/shadow check ==
  In1 : Inport
  Compare To Constant : simulink/Logic and Bit Operations/Compare To Constant  relop=<  const=0  OutDataTypeStr=boolean
  Product5 : Product
  Out1 : Outport
  wires:
  Product5/1 -> Out1/1
  In1/1 -> Compare To Constant/1, Product5/1
  Compare To Constant/1 -> Product5/2

== system simulation_with_sensors/Kinematics/Kinematics 312/Euler angles/Subsystem ==
  In1 : Inport
  In2 : Inport  Port=2
  In3 : Inport  Port=3
  Cos : Trigonometry  Operator=cos
  Product : Product
  Product1 : Product
  Sin : Trigonometry
  Sum : Sum
  Out1 : Outport
  wires:
  In3/1 -> Sin/1, Cos/1
  In1/1 -> Product/1
  Cos/1 -> Product/2
  Sin/1 -> Product1/1
  In2/1 -> Product1/2
  Product/1 -> Sum/1
  Product1/1 -> Sum/2
  Sum/1 -> Out1/1

== system simulation_with_sensors/Kinematics/Kinematics 312/Euler angles/Subsystem1 ==
  In1 : Inport
  In2 : Inport  Port=2
  In3 : Inport  Port=3
  Cos : Trigonometry  Operator=cos
  Product : Product
  Product1 : Product
  Sin : Trigonometry
  Sum : Sum
  Out1 : Outport
  wires:
  Sum/1 -> Out1/1
  Product1/1 -> Sum/2
  Product/1 -> Sum/1
  In2/1 -> Product1/2
  Sin/1 -> Product1/1
  Cos/1 -> Product/2
  In1/1 -> Product/1
  In3/1 -> Cos/1, Sin/1

== system simulation_with_sensors/Kinematics/Kinematics 312/Euler angles/Subsystem2 ==
  In1 : Inport
  In2 : Inport  Port=2
  In3 : Inport  Port=3
  Cos : Trigonometry  Operator=cos
  Product : Product
  Product1 : Product
  Sin : Trigonometry
  Sum : Sum
  Out1 : Outport
  wires:
  In3/1 -> Sin/1, Cos/1
  In1/1 -> Product/1
  Cos/1 -> Product/2
  Sin/1 -> Product1/1
  In2/1 -> Product1/2
  Product/1 -> Sum/1
  Product1/1 -> Sum/2
  Sum/1 -> Out1/1

== system simulation_with_sensors/Kinematics/Kinematics 312/s_312 - A/R1 ==
  x : Inport
  Constant : Constant  Value=[1; 0; 0]
  Constant1 : Constant  Value=0
  Cos : Trigonometry  Operator=cos
  Gain : Gain  Gain=-1
  Matrix Concatenate : Concatenate  NumInputs=3  Mode=Multidimensional array  ConcatenateDimension=2
  Sin : Trigonometry
  Vector Concatenate : Concatenate  NumInputs=3
  Vector Concatenate1 : Concatenate  NumInputs=3
  R1 : Outport
  wires:
  Matrix Concatenate/1 -> R1/1
  x/1 -> Cos/1, Sin/1
  Vector Concatenate1/1 -> Matrix Concatenate/2
  Constant/1 -> Matrix Concatenate/1
  Vector Concatenate/1 -> Matrix Concatenate/3
  Constant1/1 -> Vector Concatenate/1, Vector Concatenate1/1
  Cos/1 -> Vector Concatenate/3, Vector Concatenate1/2
  Gain/1 -> Vector Concatenate1/3
  Sin/1 -> Vector Concatenate/2, Gain/1

== system simulation_with_sensors/Kinematics/Kinematics 312/s_312 - A/R2 ==
  x : Inport
  Constant : Constant  Value=[0; 1; 0]
  Constant1 : Constant  Value=0
  Cos : Trigonometry  Operator=cos
  Gain : Gain  Gain=-1
  Matrix Concatenate : Concatenate  NumInputs=3  Mode=Multidimensional array  ConcatenateDimension=2
  Sin : Trigonometry
  Vector Concatenate : Concatenate  NumInputs=3
  Vector Concatenate1 : Concatenate  NumInputs=3
  R2 : Outport
  wires:
  Vector Concatenate/1 -> Matrix Concatenate/1
  x/1 -> Sin/1, Cos/1
  Matrix Concatenate/1 -> R2/1
  Constant/1 -> Matrix Concatenate/2
  Vector Concatenate1/1 -> Matrix Concatenate/3
  Constant1/1 -> Vector Concatenate/2, Vector Concatenate1/2
  Cos/1 -> Vector Concatenate1/3, Vector Concatenate/1
  Sin/1 -> Gain/1, Vector Concatenate/3
  Gain/1 -> Vector Concatenate1/1

== system simulation_with_sensors/Kinematics/Kinematics 312/s_312 - A/R3 ==
  x : Inport
  Constant : Constant  Value=[0; 0; 1]
  Constant1 : Constant  Value=0
  Cos : Trigonometry  Operator=cos
  Gain : Gain  Gain=-1
  Matrix Concatenate : Concatenate  NumInputs=3  Mode=Multidimensional array  ConcatenateDimension=2
  Sin : Trigonometry
  Vector Concatenate : Concatenate  NumInputs=3
  Vector Concatenate1 : Concatenate  NumInputs=3
  R3 : Outport
  wires:
  Vector Concatenate/1 -> Matrix Concatenate/1
  Sin/1 -> Vector Concatenate1/1, Gain/1
  Cos/1 -> Vector Concatenate1/2, Vector Concatenate/1
  Constant/1 -> Matrix Concatenate/3
  Gain/1 -> Vector Concatenate/2
  Vector Concatenate1/1 -> Matrix Concatenate/2
  x/1 -> Sin/1, Cos/1
  Constant1/1 -> Vector Concatenate/3, Vector Concatenate1/3
  Matrix Concatenate/1 -> R3/1

== system simulation_with_sensors/Kinematics/Kinematics 312/s_313 - A/R1 ==
  x : Inport
  Constant : Constant  Value=[1; 0; 0]
  Constant1 : Constant  Value=0
  Cos : Trigonometry  Operator=cos
  Gain : Gain  Gain=-1
  Matrix Concatenate : Concatenate  NumInputs=3  Mode=Multidimensional array  ConcatenateDimension=2
  Sin : Trigonometry
  Vector Concatenate : Concatenate  NumInputs=3
  Vector Concatenate1 : Concatenate  NumInputs=3
  R1 : Outport
  wires:
  Sin/1 -> Gain/1, Vector Concatenate/2
  Gain/1 -> Vector Concatenate1/3
  Cos/1 -> Vector Concatenate1/2, Vector Concatenate/3
  Constant1/1 -> Vector Concatenate1/1, Vector Concatenate/1
  Vector Concatenate/1 -> Matrix Concatenate/3
  Constant/1 -> Matrix Concatenate/1
  Vector Concatenate1/1 -> Matrix Concatenate/2
  x/1 -> Sin/1, Cos/1
  Matrix Concatenate/1 -> R1/1

== system simulation_with_sensors/Kinematics/Kinematics 312/s_313 - A/R3_1 ==
  x : Inport
  Constant : Constant  Value=[0; 0; 1]
  Constant1 : Constant  Value=0
  Cos : Trigonometry  Operator=cos
  Gain : Gain  Gain=-1
  Matrix Concatenate : Concatenate  NumInputs=3  Mode=Multidimensional array  ConcatenateDimension=2
  Sin : Trigonometry
  Vector Concatenate : Concatenate  NumInputs=3
  Vector Concatenate1 : Concatenate  NumInputs=3
  R3 : Outport
  wires:
  Matrix Concatenate/1 -> R3/1
  Constant1/1 -> Vector Concatenate1/3, Vector Concatenate/3
  x/1 -> Cos/1, Sin/1
  Vector Concatenate1/1 -> Matrix Concatenate/2
  Gain/1 -> Vector Concatenate/2
  Constant/1 -> Matrix Concatenate/3
  Cos/1 -> Vector Concatenate/1, Vector Concatenate1/2
  Sin/1 -> Gain/1, Vector Concatenate1/1
  Vector Concatenate/1 -> Matrix Concatenate/1

== system simulation_with_sensors/Kinematics/Kinematics 312/s_313 - A/R3_2 ==
  x : Inport
  Constant : Constant  Value=[0; 0; 1]
  Constant1 : Constant  Value=0
  Cos : Trigonometry  Operator=cos
  Gain : Gain  Gain=-1
  Matrix Concatenate : Concatenate  NumInputs=3  Mode=Multidimensional array  ConcatenateDimension=2
  Sin : Trigonometry
  Vector Concatenate : Concatenate  NumInputs=3
  Vector Concatenate1 : Concatenate  NumInputs=3
  R3 : Outport
  wires:
  Vector Concatenate/1 -> Matrix Concatenate/1
  Sin/1 -> Vector Concatenate1/1, Gain/1
  Cos/1 -> Vector Concatenate1/2, Vector Concatenate/1
  Constant/1 -> Matrix Concatenate/3
  Gain/1 -> Vector Concatenate/2
  Vector Concatenate1/1 -> Matrix Concatenate/2
  x/1 -> Sin/1, Cos/1
  Constant1/1 -> Vector Concatenate/3, Vector Concatenate1/3
  Matrix Concatenate/1 -> R3/1

== system simulation_with_sensors/Kinematics/Kinematics 313/Euler angles/Subsystem ==
  In1 : Inport
  In2 : Inport  Port=2
  In3 : Inport  Port=3
  Cos : Trigonometry  Operator=cos
  Product : Product
  Product1 : Product
  Sin : Trigonometry
  Sum : Sum
  Out1 : Outport
  wires:
  Sum/1 -> Out1/1
  Product1/1 -> Sum/2
  Product/1 -> Sum/1
  In2/1 -> Product1/2
  Sin/1 -> Product1/1
  Cos/1 -> Product/2
  In1/1 -> Product/1
  In3/1 -> Cos/1, Sin/1

== system simulation_with_sensors/Kinematics/Kinematics 313/Euler angles/Subsystem1 ==
  In1 : Inport
  In2 : Inport  Port=2
  In3 : Inport  Port=3
  Cos : Trigonometry  Operator=cos
  Product : Product
  Product1 : Product
  Sin : Trigonometry
  Sum : Sum
  Out1 : Outport
  wires:
  In3/1 -> Sin/1, Cos/1
  In1/1 -> Product/1
  Cos/1 -> Product/2
  Sin/1 -> Product1/1
  In2/1 -> Product1/2
  Product/1 -> Sum/1
  Product1/1 -> Sum/2
  Sum/1 -> Out1/1

== system simulation_with_sensors/Kinematics/Kinematics 313/Euler angles/Subsystem2 ==
  In1 : Inport
  In2 : Inport  Port=2
  In3 : Inport  Port=3
  Cos : Trigonometry  Operator=cos
  Product : Product
  Product1 : Product
  Sin : Trigonometry
  Sum : Sum
  Out1 : Outport
  wires:
  Sum/1 -> Out1/1
  Product1/1 -> Sum/2
  Product/1 -> Sum/1
  In2/1 -> Product1/2
  Sin/1 -> Product1/1
  Cos/1 -> Product/2
  In1/1 -> Product/1
  In3/1 -> Cos/1, Sin/1

== system simulation_with_sensors/Kinematics/Kinematics 313/s_312 - A/R1 ==
  x : Inport
  Constant : Constant  Value=[1; 0; 0]
  Constant1 : Constant  Value=0
  Cos : Trigonometry  Operator=cos
  Gain : Gain  Gain=-1
  Matrix Concatenate : Concatenate  NumInputs=3  Mode=Multidimensional array  ConcatenateDimension=2
  Sin : Trigonometry
  Vector Concatenate : Concatenate  NumInputs=3
  Vector Concatenate1 : Concatenate  NumInputs=3
  R1 : Outport
  wires:
  Matrix Concatenate/1 -> R1/1
  x/1 -> Cos/1, Sin/1
  Vector Concatenate1/1 -> Matrix Concatenate/2
  Constant/1 -> Matrix Concatenate/1
  Vector Concatenate/1 -> Matrix Concatenate/3
  Constant1/1 -> Vector Concatenate/1, Vector Concatenate1/1
  Cos/1 -> Vector Concatenate/3, Vector Concatenate1/2
  Gain/1 -> Vector Concatenate1/3
  Sin/1 -> Vector Concatenate/2, Gain/1

== system simulation_with_sensors/Kinematics/Kinematics 313/s_312 - A/R2 ==
  x : Inport
  Constant : Constant  Value=[0; 1; 0]
  Constant1 : Constant  Value=0
  Cos : Trigonometry  Operator=cos
  Gain : Gain  Gain=-1
  Matrix Concatenate : Concatenate  NumInputs=3  Mode=Multidimensional array  ConcatenateDimension=2
  Sin : Trigonometry
  Vector Concatenate : Concatenate  NumInputs=3
  Vector Concatenate1 : Concatenate  NumInputs=3
  R2 : Outport
  wires:
  Vector Concatenate/1 -> Matrix Concatenate/1
  x/1 -> Sin/1, Cos/1
  Matrix Concatenate/1 -> R2/1
  Constant/1 -> Matrix Concatenate/2
  Vector Concatenate1/1 -> Matrix Concatenate/3
  Constant1/1 -> Vector Concatenate/2, Vector Concatenate1/2
  Cos/1 -> Vector Concatenate1/3, Vector Concatenate/1
  Sin/1 -> Gain/1, Vector Concatenate/3
  Gain/1 -> Vector Concatenate1/1

== system simulation_with_sensors/Kinematics/Kinematics 313/s_312 - A/R3 ==
  x : Inport
  Constant : Constant  Value=[0; 0; 1]
  Constant1 : Constant  Value=0
  Cos : Trigonometry  Operator=cos
  Gain : Gain  Gain=-1
  Matrix Concatenate : Concatenate  NumInputs=3  Mode=Multidimensional array  ConcatenateDimension=2
  Sin : Trigonometry
  Vector Concatenate : Concatenate  NumInputs=3
  Vector Concatenate1 : Concatenate  NumInputs=3
  R3 : Outport
  wires:
  Vector Concatenate/1 -> Matrix Concatenate/1
  Sin/1 -> Vector Concatenate1/1, Gain/1
  Cos/1 -> Vector Concatenate1/2, Vector Concatenate/1
  Constant/1 -> Matrix Concatenate/3
  Gain/1 -> Vector Concatenate/2
  Vector Concatenate1/1 -> Matrix Concatenate/2
  x/1 -> Sin/1, Cos/1
  Constant1/1 -> Vector Concatenate/3, Vector Concatenate1/3
  Matrix Concatenate/1 -> R3/1
